simulink model "Final_sim"  (R2024b)
settings: Solver=VariableStepAuto  StartTime=0.0  StopTime=total_time  RelTol=1e-3
undefined symbols (not defined in the file): D, d, d_nom, ekf_online, kf, ki, P_INIT_EKF, path, prob_gps_loss, qf, qi, r, R_2, R_3, R_4, R_5, r_nom, T_s, Ta, Tc, total_time, Ts, w_max, X, Y, Z_INIT_EKF
libraries: robotlib x4
settings Model: Creator=riccardo01  LastModifiedBy=leontecosm

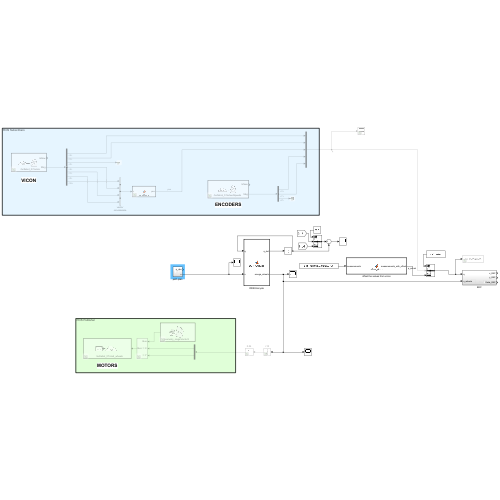
[thumbnail: Simulink's stored preview of the top-level diagram]
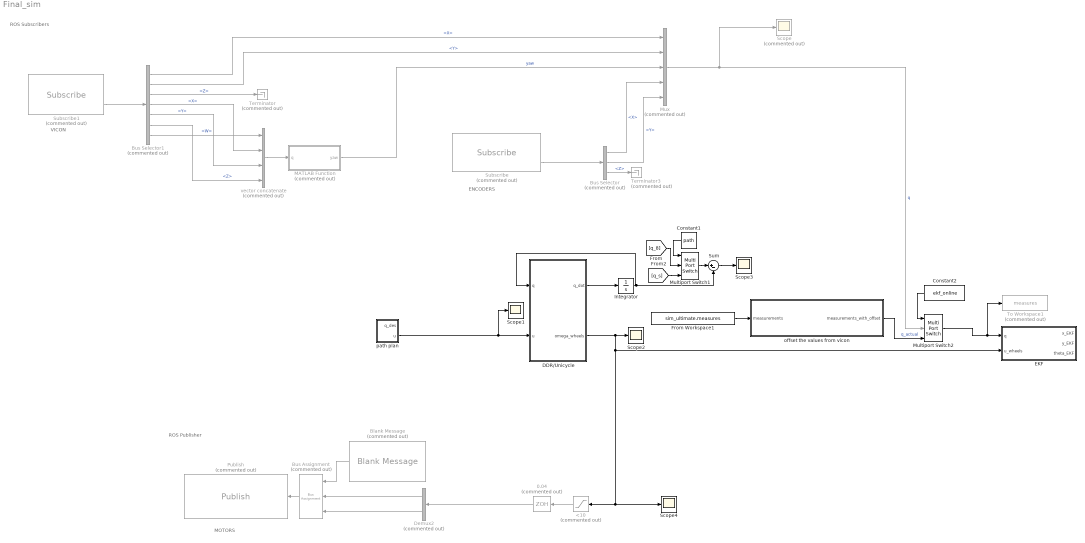
== system Final_sim ==
  note: MOTORS
  note: ROS Publisher
  note: ENCODERS
  note: VICON
  note: ROS Subscribers
  0.04 : ZeroOrderHold  Commented=on  SampleTime=Ts
  <10 : Saturate  Commented=on  UpperLimit=w_max  LowerLimit=-w_max
  Blank Message : robotlib/Blank Message  Commented=on  messageClass=Message  entityType=geometry_msgs/Vector3  messageType=geometry_msgs/Vector3  SampleTime=Ts  legacyBusStruct=off
      settings: LibrarySourceBlock=roslib/ROS/Blank Message
  Bus Assignment : BusAssignment  Commented=on  AssignedSignals=X,Y
  Bus Selector : BusSelector  Commented=on  OutputSignals=X,Y,Z
  Bus Selector1 : BusSelector  Commented=on  OutputSignals=Pose.Pose.Position.X,Pose.Pose.Position.Y,Pose.Pose.Position.Z,Pose.Pose.Orientation.X,Pose.Pose.Orientation.Y,Pose.Pose.Orientation.Z,Pose.Pose.Orientation.W
  Constant1 : Constant  Value=path
  Constant2 : Constant  Value=ekf_online
  DDR/Unicycle : MATLAB Function  TreatAsAtomicUnit=on
  Demux2 : Demux  Commented=on  Outputs=2
  EKF : Subsystem
  From Workspace1 : FromWorkspace  VariableName=sim_ultimate.measures
  Integrator : Integrator  InitialCondition=[0,0,0]'
  MATLAB Function : MATLAB Function  Commented=on  TreatAsAtomicUnit=on
  Multiport Switch1 : MultiPortSwitch  Inputs=2  SaturateOnIntegerOverflow=off  InputSameDT=off
  Multiport Switch2 : MultiPortSwitch  Inputs=2  SaturateOnIntegerOverflow=off  InputSameDT=off
  Mux : Mux  Commented=on  Inputs=5
  Publish : robotlib/Publish  Commented=on  topicSource=Specify your own  topic=/turtlebot_07/cmd_wheels  messageType=geometry_msgs/Vector3  legacyBusStruct=off  messageQueueLength=1
      settings: LibrarySourceBlock=roslib/ROS/Publish
  Scope : Scope  Commented=on
  Scope{1..4} (4 alike) : Scope
  Subscribe : robotlib/Subscribe  Commented=on  topicSource=Specify your own  topic=/turtlebot_07/wheelSpeeds  messageType=geometry_msgs/Vector3  SampleTime=-1  legacyBusStruct=off  messageQueueLength=1
      settings: LibrarySourceBlock=roslib/ROS/Subscribe
  Subscribe1 : robotlib/Subscribe  Commented=on  topicSource=Specify your own  topic=/turtlebot_07/odom  messageType=nav_msgs/Odometry  SampleTime=-1  legacyBusStruct=off  messageQueueLength=1
      settings: LibrarySourceBlock=roslib/ROS/Subscribe
  Sum : Sum  Inputs=|+-
  Terminator : Terminator  Commented=on
  Terminator3 : Terminator  Commented=on
  To Workspace1 : ToWorkspace  Commented=on  VariableName=measures  SaveFormat=Structure With Time  SampleTime=-1
  offset the values from vicon : MATLAB Function  TreatAsAtomicUnit=on
  path plan : Subsystem
  vector concatenate : Concatenate  Commented=on  NumInputs=4
  wires:
  DDR/Unicycle/1(q_dot) -> Integrator/1
  Integrator/1 -> DDR/Unicycle/1(q), Sum/2
  Sum/1 -> Scope3/1
  0.04/1 -> Demux2/1
  Blank Message/1 -> Bus Assignment/1
  <10/1 -> 0.04/1
  Demux2/2 -> Bus Assignment/3
  Bus Assignment/1 -> Publish/1
  Demux2/1 -> Bus Assignment/2
  DDR/Unicycle/2(omega_wheels) -> <10/1, Scope4/1, EKF/2(u_wheels), Scope2/1
  vector concatenate/1 -> MATLAB Function/1(q)
  Subscribe/2 -> Bus Selector/1
  Bus Selector1/5 -> vector concatenate/3  "<Y>"
  Bus Selector/2 -> Mux/5  "<Y>"
  Bus Selector1/3 -> Terminator/1  "<Z>"
  Bus Selector1/1 -> Mux/1  "<X>"
  MATLAB Function/1(yaw) -> Mux/3  "yaw"
  Subscribe1/2 -> Bus Selector1/1
  Bus Selector1/6 -> vector concatenate/4  "<Z>"
  Bus Selector/1 -> Mux/4  "<X>"
  Mux/1 -> Scope/1, Multiport Switch2/2  "q"
  Bus Selector/3 -> Terminator3/1  "<Z>"
  Bus Selector1/2 -> Mux/2  "<Y>"
  Bus Selector1/7 -> vector concatenate/1  "<W>"
  Bus Selector1/4 -> vector concatenate/2  "<X>"
  path plan/2(u) -> Scope1/1, DDR/Unicycle/2(u)
  Constant1/1 -> Multiport Switch1/1
  Multiport Switch1/1 -> Sum/1
  [q_8] -> Multiport Switch1/2
  [q_s] -> Multiport Switch1/3
  From Workspace1/1 -> offset the values from vicon/1(measurements)
  Multiport Switch2/1 -> To Workspace1/1, EKF/1(q)
  offset the values from vicon/1(measurements_with_offset) -> Multiport Switch2/3  "q_actual"
  Constant2/1 -> Multiport Switch2/1

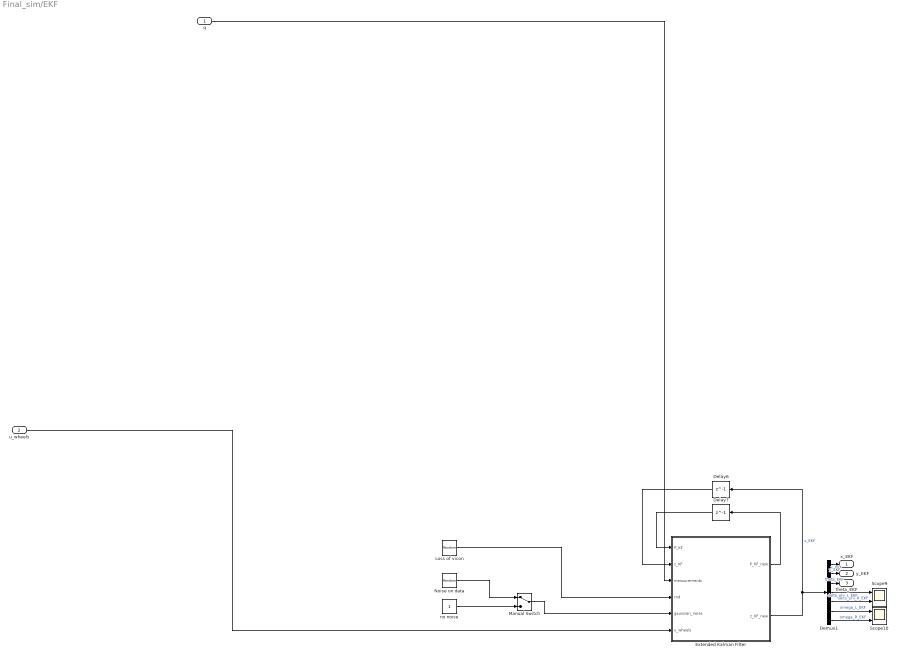
== system Final_sim/EKF ==
  q : Inport
  u_wheels : Inport  Port=2
  " Loss of vicon" : UniformRandomNumber  Minimum=0
  Delay6 : Delay  DelayLength=1  InitialCondition=Z_INIT_EKF
  Delay7 : Delay  DelayLength=1  InitialCondition=P_INIT_EKF
  Demux1 : Demux  Outputs=7
  Extended Kalman Filter : MATLAB Function  TreatAsAtomicUnit=on
  Manual Switch : ManualSwitch
  Noise on data : RandomNumber  Variance=0.0001
  Scope10 : Scope  NumInputPorts=2
  Scope9 : Scope  NumInputPorts=2
  no noise : Constant
  x_EKF : Outport
  y_EKF : Outport  Port=2
  theta_EKF : Outport  Port=3
  wires:
  Demux1/6 -> Scope10/1  "omega_L_EKF"
  Demux1/3 -> theta_EKF/1  "theta_EKF"
  Delay6/1 -> Extended Kalman Filter/2(z_KF)
  Delay7/1 -> Extended Kalman Filter/1(P_KF)
  Noise on data/1 -> Manual Switch/1
  Demux1/5 -> Scope9/2  "delta_phi_R_EKF"
  Demux1/7 -> Scope10/2  "omega_R_EKF"
  Extended Kalman Filter/1(P_KF_new) -> Delay7/1
  Manual Switch/1 -> Extended Kalman Filter/5(gaussian_noise)
  " Loss of vicon"/1 -> Extended Kalman Filter/4(rnd)
  Demux1/1 -> x_EKF/1  "x_EKF"
  Demux1/4 -> Scope9/1  "delta_phi_L_EKF"
  no noise/1 -> Manual Switch/2
  u_wheels/1 -> Extended Kalman Filter/6(u_wheels)
  Extended Kalman Filter/2(z_KF_new) -> Demux1/1, Delay6/1  "z_EKF"
  q/1 -> Extended Kalman Filter/3(messurements)
  Demux1/2 -> y_EKF/1  "y_EKF"

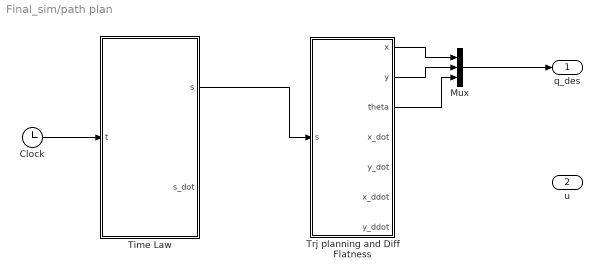
== system Final_sim/path plan ==
  Clock : Clock
      settings: Decimation=1/Ts
  Mux : Mux  Inputs=3
  Time Law : MATLAB Function  TreatAsAtomicUnit=on
  Trj planning and Diff Flatness : MATLAB Function  TreatAsAtomicUnit=on
  q_des : Outport
  u : Outport  Port=2
  wires:
  Clock/1 -> Time Law/1(t)
  Time Law/1(s) -> Trj planning and Diff Flatness/1(s)
  Trj planning and Diff Flatness/1(x) -> Mux/1
  Trj planning and Diff Flatness/2(y) -> Mux/2
  Trj planning and Diff Flatness/3(theta) -> Mux/3
  Mux/1 -> q_des/1

== matlab function Final_sim/DDR//Unicycle ==
  data: q input; u input; q_dot output; omega_wheels output; d_nom parameter; r_nom parameter
function [q_dot, omega_wheels] = DDR_Unicycle(q, u, d_nom, r_nom)
v = u(1);
omega = u(2);

q_dot = [cos(q(3))*v; sin(q(3))*v; omega];

%evaluation of speed wheels
omega_L = (2*v - d_nom*omega) / (2*r_nom);
omega_R = (2*v + d_nom*omega) / (2*r_nom);
omega_wheels=[omega_R; omega_L];

== matlab function Final_sim/path plan/Time Law ==
  data: t input; s output; s_dot output; total_time parameter; Ta parameter; Tc parameter
function [s, s_dot] = fcn(t,total_time,Ta, Tc)
s=0;
s_dot=0;

Vc=1/(Ta+Tc);% velocità costante
a=Vc/Ta;% acceleration

switch 1 %formula on the slide
    case t<Ta
        s_dot=a*t;
        s=(a*(t^2))/2;

    case (t>=Ta)&&(t<(Tc+Ta))
        s_dot=Vc;
        s=(a*(Ta^2))/2+Vc*(t-Ta);

    case (t>=(Tc+Ta))&&(t<(Tc+2*Ta))
        s_dot=Vc-a*(t-Ta-Tc);
        s=(a*(Ta^2))/2+Vc*Tc+Vc*(t-Ta-Tc)-a*(t-Ta-Tc)^2/2;

    case t>=(Tc+2*Ta)
        s_dot=0;
        s=1;


end

== matlab function Final_sim/path plan/Trj planning and Diff Flatness ==
  data: x output; y output; theta output; qi parameter; qf parameter; s input; x_dot output; y_dot output; x_ddot output; y_ddot output; ki parameter; kf parameter
function [x, y,theta,x_dot,y_dot,x_ddot,y_ddot] =Path_planning_cartesian(qi, qf, s, ki, kf)
    % s as vector like 0:0.1:1000
    %evaluate the weight as written in the slide
    a1 = qf(1);
    a2 = qi(1);
    b1 = qf(2);
    b2 = qi(2);
    
    a4 = ki*cos(qi(3)) + 3*qi(1);
    a3 = kf*cos(qf(3)) - 3*qf(1);
    
    b4 = ki*sin(qi(3)) + 3*qi(2);
    b3 = kf*sin(qf(3)) - 3*qf(2);
    
    % evaluate path
    x = a1*s.^3 - a2*(s-1).^3 + a3*s.^2.*(s-1) + a4*s.*(s-1).^2;
    y = b1*s.^3 - b2*(s-1).^3 + b3*s.^2.*(s-1) + b4*s.*(s-1).^2;

    %analitical calculation of velocity
    x_dot=3*a1*s.^2-3*a2*(s-1).^2+a3*(2*s.*(s-1)+s.^2)+a4*((s-1).^2+s.*2.*(s-1));
    y_dot=3*b1*s.^2-3*b2*(s-1).^2+b3*(2*s.*(s-1)+s.^2)+b4*((s-1).^2+s.*2.*(s-1));

    %analitical calculation of acceleration
    x_ddot=6*a1*s-6*a2*(s-1)+a3*(2*s+2*(s+(s-1)))+a4*(2*(s-1)+2*((s-1)+s));
    y_ddot=6*b1*s-6*b2*(s-1)+b3*(2*s+2*(s+(s-1)))+b4*(2*(s-1)+2*((s-1)+s));
    
    theta = atan2(y_dot, x_dot);
    
    v = sqrt(y_dot^2 +  x_dot^2);
    omega = (x_dot*y_ddot - y_dot*x_ddot)/(y_dot^2 +  x_dot^2);

end

== matlab function Final_sim/offset the values from vicon ==
  data: measurements input; measurements_with_offset output; Q_INIT parameter
function measurements_with_offset  = offset_vicon(measurements, Q_INIT)

persistent initial_vicon_pose;
persistent first_run;

% Record first vicon measurement as reference and use it for offset
if isempty(first_run)
    first_run = false;
    initial_vicon_pose = [measurements(1); measurements(2); measurements(3)];
end

% relative transformation from initial vicon pose
delta_x     = measurements(1) - initial_vicon_pose(1);
delta_y     = measurements(2) - initial_vicon_pose(2);
delta_angle = measurements(3) - initial_vicon_pose(3);


% rotation matrix to account for angle offset
rot_matrix = [cos(Q_INIT(3)), -sin(Q_INIT(3));
              sin(Q_INIT(3)),  cos(Q_INIT(3))];

% transform position
rotated_xy = rot_matrix * [delta_x; delta_y];

% fliping the theta because it shows wrong
delta_angle = -delta_angle;
rotated_xy(1) = -rotated_xy(1);

measurements_with_offset = measurements;
measurements_with_offset(1) = Q_INIT(1) + rotated_xy(1);
measurements_with_offset(2) = Q_INIT(2) + rotated_xy(2);
measurements_with_offset(3) = Q_INIT(3) + delta_angle;
end

== matlab function Final_sim/EKF/Extended Kalman Filter ==
  data: P_KF input; P_KF_new output; z_KF input; messurements input; D parameter; R_2 parameter; R_3 parameter; R_4 parameter; R_5 parameter; T_s parameter; r parameter; d parameter; prob_gps_loss parameter; rnd input; gaussian_noise input; z_KF_new output; u_wheels input
function [P_KF_new, z_KF_new] = EKF_filtering(P_KF, z_KF, messurements, D, R_2, R_3, R_4, R_5 ,T_s, r, d, prob_gps_loss, rnd, gaussian_noise,u_wheels)

% z_KF = [x_EKF, y_EKF, theta_EKF, delta_phi_L_EKF, delta_phi_R_EKF, omega_L_EKF, omega_R_EKF]

v_k = r * (z_KF(6) + z_KF(7))/2;
w_k = r * (z_KF(7) - z_KF(6))/d;

theta_mean = z_KF(3) + (w_k * T_s)/2;

F_k = [1, 0, -T_s * v_k * sin(theta_mean), 0, 0, T_s * r * cos(theta_mean)/2 + (T_s)^2 * r * v_k * sin(theta_mean)/(2*d), T_s * r * cos(theta_mean)/2 - (T_s)^2 * r * v_k * sin(theta_mean)/(2*d);
    0, 1, T_s * v_k * cos(theta_mean), 0, 0, T_s * r * sin(theta_mean)/2 - (T_s)^2 * r * v_k * cos(theta_mean)/(2*d), T_s * r * sin(theta_mean)/2 + (T_s)^2 * r * v_k * cos(theta_mean)/(2*d);
    0, 0, 1, 0, 0, (-T_s*r)/d, (T_s*r)/d;
    0, 0, 0, 0, 0, T_s, 0;
    0, 0, 0, 0, 0, 0, T_s;
    0, 0, 0, 0, 0, 0, 0;
    0, 0, 0, 0, 0, 0, 0];

%% Prediction part

z_pred = [z_KF(1)+(T_s*r*(z_KF(6)+z_KF(7))/2)*cos(theta_mean + (T_s*r*(z_KF(6)+z_KF(7)))/(2*d));
    z_KF(2)+(T_s*r*(z_KF(6)+z_KF(7))/2)*sin(theta_mean + (T_s*r*(z_KF(7)-z_KF(6)))/(2*d));
    theta_mean + (T_s*r*(z_KF(7)-z_KF(6))/(2*d));
    T_s*z_KF(6);
    T_s*z_KF(7);
    u_wheels(1);
    u_wheels(2)];

P_pred = F_k * P_KF * F_k' + D;


%% Update

if(rnd<prob_gps_loss) 

    % Just encoders
    y_messurement = [messurements(1); messurements(2)];
    H = [0, 0, 0, 1, 0, 0, 0;
        0, 0, 0, 0, 1, 0, 0];

    e = y_messurement - H * z_pred;
    K = P_pred * H' /(H * P_pred * H' + R_2);

    z_KF_new = z_pred +  K * e;
    P_KF_new = P_pred - K * H * P_pred;

else 
    % GPS(x,y,yaw) + Encoders(omegaL,omegaR)
    y_messurement = [messurements(3)+gaussian_noise;messurements(4)+gaussian_noise; messurements(1); messurements(2)];

    H = [1, 0, 0, 0, 0, 0, 0;
         0, 1, 0, 0, 0, 0, 0;
         0, 0, 1, 0, 0, 0, 0;
         0, 0, 0, 0, 0, 1, 0;
         0, 0, 0, 0, 0, 0, 1];

    e = y_messurement - H * z_pred;
    K = P_pred * H' /(H * P_pred * H' + R_5);

    z_KF_new = z_pred + K * e;
    P_KF_new = P_pred - K * H * P_pred;

end

== matlab function Final_sim/MATLAB Function ==
  data: q input; yaw output
function yaw = quat2yaw(q)

% normalize to avoid issues
q = q / norm(q);

w = q(1);
x = q(2);
y = q(3);
z = q(4);

% rotation around Z axis
yaw = atan2(2*(w*z + x*y), 1 - 2*(y^2 + z^2));

end
